simulink model "generateTraj"  (R2016b)
settings: Solver=FixedStepAuto  StartTime=0.0  StopTime=330  FixedStep=0.001  RelTol=1e-3  EnableMultiTasking=on
undefined symbols (not defined in the file or in its folder): sigbuilder_block
settings Model: Creator=Vaibhav Gupta  LastModifiedBy=gupta
settings DataIOCC: LimitDataPoints=on  SaveFormat=Array
settings OptimizationCC: LifeSpan=inf
settings DebuggingCC: SFUnexpectedBacktrackingDiag=warning  SFNoUnconditionalDefaultTransitionDiag=warning  SFExecutionAtInitializationDiag=none
settings HardwareCC: ProdBitPerPointer=32  ProdBitPerSizeT=32  ProdBitPerPtrDiffT=32  ProdLargestAtomicFloat=None  ProdIntDivRoundTo=Undefined  ProdEndianess=Unspecified  ProdWordSize=32  ProdHWDeviceType=32-bit Generic
settings ModelReferenceCC: PropagateSignalLabelsOutOfModel=off
settings GRTTargetCC: TargetLangStandard=C89/C90 (ANSI)  GeneratePreprocessorConditionals=Disable all
settings ConfigComp: CovMetricSettings=dw  CovHtmlReporting=on  CovSaveCumulativeToWorkspaceVar=on  CovSaveSingleToWorkspaceVar=on  CovExternalEMLEnable=off

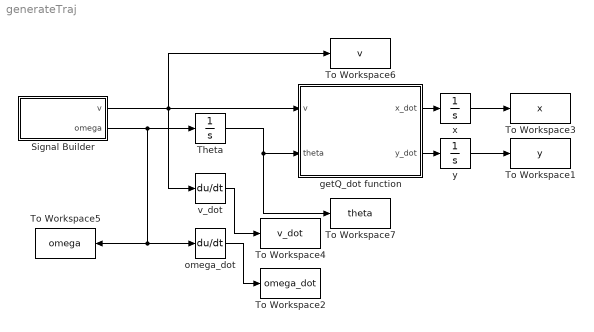
== system generateTraj ==
  Signal Builder : Subsystem  Tag=STV Subsys  LoadFcn=sigbuilder_block('load',[6 30 1012.5 447.75 ]);  StartFcn=sigbuilder_block('start');  StopFcn=sigbuilder_block('stop');  ClipboardFcn=sigbuilder_block('clipboard');  mask(Sigbuilder block){tuvar=[0:10]}
      mask help: Simulink:masks:SigbuilderBlock_MD
      mask init:
      | if ~strcmp(get_param(bdroot(gcbh),'SimulationStatus'),'stopped') tuvar = sigbuilder_block('maskInit'); end
      settings: CopyFcn=sigbuilder_block('copy');  DeleteFcn=sigbuilder_block('delete');  ModelCloseFcn=sigbuilder_block('modelClose');  PreSaveFcn=sigbuilder_block('preSave');  PauseFcn=sigbuilder_block('pause');  ContinueFcn=sigbuilder_block('continue');  NameChangeFcn=sigbuilder_block('namechange');  OpenFcn=sigbuilder_block('open',[6 30 1012.5 447.75 ]);  CloseFcn=sigbuilder_block('close');
      mask Display: plot(0, 0, 100, 100,[2, 2, 32, 32, 2], [68, 8, 8, 68, 68],[32, 2], [38, 38], [32, 19, 2],[53, 60, 44], [32, 17, 17, 2],[16, 16, 31, 31]);txt = getActiveGroup(gcbh);text(2, 100, txt,'verticalAlignment', 'top');
  Theta : Integrator  InitialCondition=pi/2
  To Workspace1 : ToWorkspace  VariableName=y  SaveFormat=Structure With Time  SampleTime=0.001
      settings: Decimation=2
  To Workspace2 : ToWorkspace  VariableName=omega_dot  SaveFormat=Structure With Time  SampleTime=0.001
      settings: Decimation=2
  To Workspace3 : ToWorkspace  VariableName=x  SaveFormat=Structure With Time  SampleTime=0.001
      settings: Decimation=2
  To Workspace4 : ToWorkspace  VariableName=v_dot  SaveFormat=Structure With Time  SampleTime=0.001
      settings: Decimation=2
  To Workspace5 : ToWorkspace  VariableName=omega  SaveFormat=Structure With Time  SampleTime=0.001
      settings: Decimation=2
  To Workspace6 : ToWorkspace  VariableName=v  SaveFormat=Structure With Time  SampleTime=0.001
      settings: Decimation=2
  To Workspace7 : ToWorkspace  VariableName=theta  SaveFormat=Structure With Time  SampleTime=0.001
      settings: Decimation=2
  getQ_dot function : MATLAB Function  TreatAsAtomicUnit=on
  omega_dot : Derivative  CoefficientInTFapproximation=0
  v_dot : Derivative  CoefficientInTFapproximation=0
  x : Integrator  InitialCondition=500
  y : Integrator
  wires:
  Signal Builder/2(omega) -> Theta/1, To Workspace5/1, omega_dot/1
  Signal Builder/1(v) -> To Workspace6/1, v_dot/1, getQ_dot function/1(v)
  getQ_dot function/1(x_dot) -> x/1
  getQ_dot function/2(y_dot) -> y/1
  x/1 -> To Workspace3/1
  y/1 -> To Workspace1/1
  omega_dot/1 -> To Workspace2/1
  v_dot/1 -> To Workspace4/1
  Theta/1 -> To Workspace7/1, getQ_dot function/2(theta)

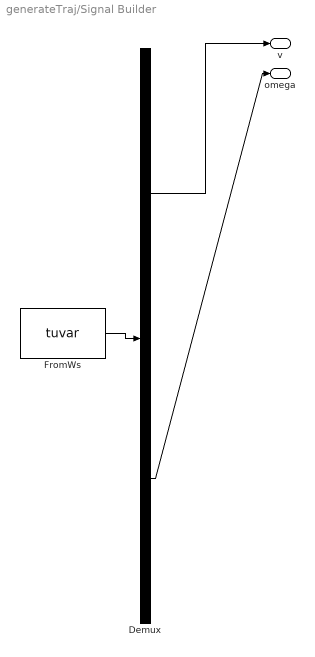
== system generateTraj/Signal Builder ==
  Demux : Demux  Tag=STV Demux  Outputs=2
  FromWs : FromWorkspace  Tag=STV FromWs  VariableName=tuvar  SampleTime=0  OutputAfterFinalValue=Holding final value
      SigBuilderData=|
      | common.afterFinalStr = 'Hold final value'
      | common.sampleTime = '0'
      | dataSet.timeRange = [0 330]
      | dataSet.name = 'Group 1'
      | sbobj.Groups.Name = 'Group 1'
      | sbobj.Groups.Signals(1).Name = 'v'
      | sbobj.Groups.Signals(1).XData = [0 10 20 30 60 70 100 110 140 150 180 190 220 230 260 270 300 310 320 330]
      | sbobj.Groups.Signals(1).YData = [0 25 25 0 0 25 25 0 0 25 25 0 0 25 25 0 0 25 25 0]
      | sbobj.Groups.Signals(2).Name = 'omega'
      | sbobj.Groups.Signals(2).XData = [0 30 40 50 60 110 120 130 140 190 200 210 220 270 280 290 300 330]
      | sbobj.Groups.Signals(2).YData = [0 0 0.0785 0.0785 0 0 0.0785 0.0785 0 0 0.0785 0.0785 0 0 0.0785 0.0785 0 0]
      | sbobj.Groups.TimeRange = [0 330]
  v : Outport  Tag=STV Outport
  omega : Outport  Tag=STV Outport  Port=2
  wires:
  Demux/1 -> v/1
  FromWs/1 -> Demux/1
  Demux/2 -> omega/1

== matlab function generateTraj/getQ_dot function ==
  data: v input; theta input; x_dot output; y_dot output
function [x_dot, y_dot] = getQ_dot(v, theta)
%% getTorque
% This gives the required value of torque for the motion

sTheta = sin(theta);
cTheta = cos(theta);

x_dot = v * cTheta;
y_dot = v * sTheta;
